simulink model "lokta_volterra"  (R2020b)
settings: Solver=VariableStepAuto  StartTime=0.0  StopTime=100.0  RelTol=1e-3
settings Model: Creator=SOFIACRISTINADURANMU  LastModifiedBy=SOFIACRISTINADURANMU
settings DataIOCC: ReturnWorkspaceOutputs=off  TimeSaveName=t

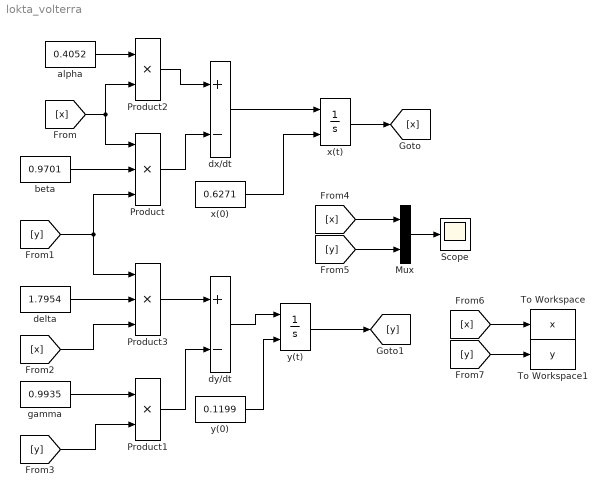
== system lokta_volterra ==
  Mux : Mux  Inputs=2
  Product : Product  Inputs=3
  Product1 : Product
  Product2 : Product
  Product3 : Product  Inputs=3
  Scope : Scope
  To Workspace : ToWorkspace  VariableName=x  SampleTime=-1
  To Workspace1 : ToWorkspace  VariableName=y  SampleTime=-1
  alpha : Constant  Value=0.4052
  beta : Constant  Value=0.9701
  delta : Constant  Value=1.7954
  dx/dt : Sum  Inputs=+-
  dy/dt : Sum  Inputs=+-
  gamma : Constant  Value=0.9935
  x(0) : Constant  Value=0.6271
  x(t) : Integrator  InitialConditionSource=external
  y(0) : Constant  Value=0.1199
  y(t) : Integrator  InitialConditionSource=external
  wires:
  Product2/1 -> dx/dt/1
  Product/1 -> dx/dt/2
  x(t)/1 -> [x]
  [x] -> Product2/2, Product/1
  x(0)/1 -> x(t)/2
  dx/dt/1 -> x(t)/1
  alpha/1 -> Product2/1
  beta/1 -> Product/2
  [y] -> Product/3, Product3/1
  Product3/1 -> dy/dt/1
  delta/1 -> Product3/2
  [x] -> Product3/3
  gamma/1 -> Product1/1
  [y] -> Product1/2
  Product1/1 -> dy/dt/2
  dy/dt/1 -> y(t)/1
  y(0)/1 -> y(t)/2
  y(t)/1 -> [y]
  [x] -> Mux/1
  [y] -> Mux/2
  Mux/1 -> Scope/1
  [x] -> To Workspace/1
  [y] -> To Workspace1/1
